simulink model "ServoCalibration"  (R2021b)
settings: Solver=FixedStepAuto  StartTime=0.0  StopTime=600  RelTol=1e-3  EnableMultiTasking=on
InitFcn:
  | hardwareSetup;
model workspace (MAT data in the model file):
  Ts_DynSim = Simulink.Parameter
  Ts_DynSim.Value = 0.005
  Ts_DynSim.DataType = 'auto'
  Ts_DynSim.Complexity = 'real'
  Ts_DynSim.Dimensions = [1 1]
values from neighbouring files (symbols this model uses):
  Ts_DynSim = 0.005    [MPCGen_OffsetFree.m]    (also in MPCGen_OffsetFree_UD.m; MPCGen_OffsetFree_estDis.m = 0.006; MPCcontrollerGen_OffsetFree.m; MPCcontrollerGen_OffsetFree_UD.m)
libraries: PuppyLibrary x5, simulink_extras x2
settings Model: SimulationMode=external  ExtModeTrigDuration=2  Creator=MSI-NB  LastModifiedBy=MSI-NB
settings SolverCC: AlgebraicLoopSolver=TrustRegion  PositivePriorityOrder=on
settings DataIOCC: ReturnWorkspaceOutputs=off
settings OptimizationCC: MaxStackSize=64
settings DebuggingCC: ParameterTunabilityLossMsg=error  SFMachineParentedDataDiag=warning  ArithmeticOperatorsInVariantConditions=warning
settings HardwareCC: ProdBitPerPointer=32  ProdBitPerSizeT=32  ProdBitPerPtrDiffT=32  ProdLargestAtomicInteger=Long  ProdLargestAtomicFloat=Double  ProdWordSize=32  ProdHWDeviceType=ARM Compatible->ARM Cortex  UseEmbeddedCoderFeatures=off
settings SFSimCC: SimUseLocalCustomCode=off  CustomCodeUndefinedFunction=UseInterfaceOnly
settings RTWCC: Description=Embedded Coder  SystemTargetFile=ert.tlc  HardwareBoard=Raspberry Pi  TLCOptions="-aInlineSetEventsForThisBaseRateFcn=TLC_FALSE -aSuppressMultiTaskScheduler=TLC_FALSE  -aRateBasedStepFcn=0"  TemplateMakefile=ert_default_tmf  RTWUseLocalCustomCode=off  Toolchain=GNU GCC Embedded Linux  BuildConfiguration=Faster Runs
settings CodeAppCC: ForceParamTrailComments=on  OperatorAnnotations=on  StateflowObjectComments=on  MATLABSourceComments=on
settings ERTTargetCC: ERTCustomFileBanners=off  SupportContinuousTime=on  SupportNonInlinedSFcns=on  RemoveResetFunc=off  SupportVariableSizeSignals=on  ModelStepFunctionPrototypeControlCompliant=off

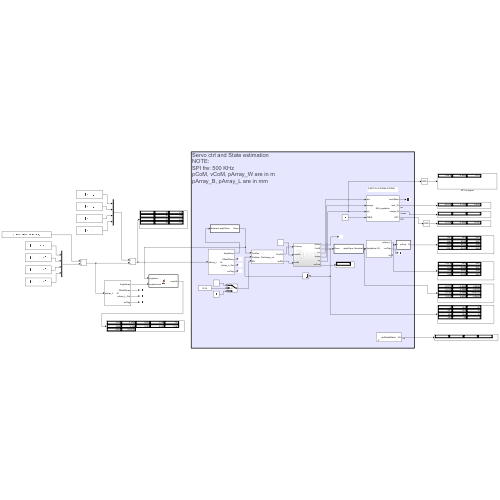
[thumbnail: Simulink's stored preview of the top-level diagram]
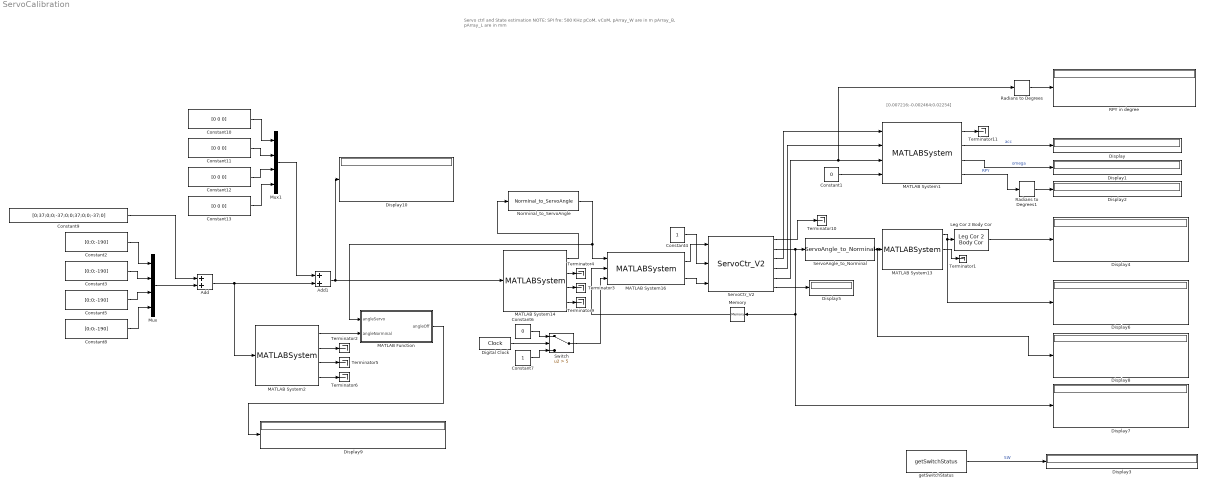
== system ServoCalibration ==
  note: [0.007216;-0.002464;0.02254]
  note: Servo ctrl and State estimation
      | NOTE:
      | SPI fre: 500 KHz
      | pCoM, vCoM, pArray_W are in m
      | pArray_B, pArray_L are in mm
  Add : Sum
  Add1 : Sum
  Constant1 : Constant  Value=0
  Constant{10..13} (4 alike) : Constant  Value=[0 0 0]
  Constant{2..3,5,8} (4 alike) : Constant  Value=[0;0;-190]
  Constant4 : Constant
  Constant6 : Constant  Value=0
  Constant7 : Constant
  Constant9 : Constant  Value=[0;37;0;0;-37;0;0;37;0;0;-37;0]
  Digital Clock : DigitalClock  SampleTime=Ts_DynSim
  Display{,1..10} (11 alike) : Display
  Leg Cor 2 Body Cor : PuppyLibrary/Leg Cor 2 Body Cor  SystemSampleTime=-1  VariantActivationTime=update diagram  Latency=0  AutoFrameSizeCalculation=off
  MATLAB Function : MATLAB Function  TreatAsAtomicUnit=on
  MATLAB System1 : MATLABSystem  System=IMU_regulation  pitOff=-0.4  rollOff=1  SimulateUsing=Code generation
      mask Type: IMU_regulation
      mask Display:
      | disp('IMU_regulation');
      | port_label('input',1,'acc');
      | port_label('input',2,'omega');
      | port_label('input',3,'rpy');
      | port_label('input',4,'OffEN');
      | port_label('output',1,'accOffnow');
      | port_label('output',2,'accL_W');
      | port_label('output',3,'omega_W');
      | port_label('output',4,'RPY');
  MATLAB System13 : MATLABSystem  System=FK  dt=0.005  SimulateUsing=Code generation
      mask Type: FK
      mask Display:
      | disp('FK');
      | port_label('input',1,'AngleArray');
      | port_label('output',1,'pArray_L');
      | port_label('output',2,'errFlag');
      | port_label('output',3,'dq');
  MATLAB System14 : MATLABSystem  System=IK  LF_Off=[ 0; 0; 0 ]  RF_Off=[ 0; 0; 0 ]  LH_Off=[ 0; 0; 0 ]  RH_Off=[ 0; 0; 0 ]  SimulateUsing=Code generation
      mask Type: IK
      mask Display:
      | disp('IK');
      | port_label('input',1,'pArray_L');
      | port_label('output',1,'AngleArray');
      | port_label('output',2,'OffsetPArray');
      | port_label('output',3,'pArray_L_Out');
      | port_label('output',4,'errFlag');
  MATLAB System16 : MATLABSystem  System=PosAssign_vel  cons_Vel=15  dt=Ts_DynSim  SimulateUsing=Code generation
      mask Type: PosAssign_vel
      mask Display:
      | disp('PosAssign_vel');
      | port_label('input',1,'PosDes');
      | port_label('input',2,'PosNow');
      | port_label('input',3,'EN');
      | port_label('output',1,'PosOut');
      | port_label('output',2,'setEN');
  MATLAB System2 : MATLABSystem  System=IK  LF_Off=[ 0; 0; 0 ]  RF_Off=[ 0; 0; 0 ]  LH_Off=[ 0; 0; 0 ]  RH_Off=[ 0; 0; 0 ]  SimulateUsing=Code generation
      mask Type: IK
      mask Display:
      | disp('IK');
      | port_label('input',1,'pArray_L');
      | port_label('output',1,'AngleArray');
      | port_label('output',2,'OffsetPArray');
      | port_label('output',3,'pArray_L_Out');
      | port_label('output',4,'errFlag');
  Memory : Memory  InitialCondition=zeros(12,1)
  Mux : Mux
  Mux1 : Mux
  Norminal_to_ServoAngle : PuppyLibrary/Norminal_to_ServoAngle  SystemSampleTime=-1  VariantActivationTime=update diagram  Latency=0  AutoFrameSizeCalculation=off
  RPY in degree : Display
  Radians to Degrees : simulink_extras/Transformations/Radians to Degrees
  Radians to Degrees1 : simulink_extras/Transformations/Radians to Degrees
  ServoAngle_to_Norminal : PuppyLibrary/ServoAngle_to_Norminal  SystemSampleTime=-1  VariantActivationTime=update diagram  Latency=0  AutoFrameSizeCalculation=off
  ServoCtr_V2 : PuppyLibrary/ServoCtr_V2  SystemSampleTime=-1  VariantActivationTime=update diagram  Latency=0  AutoFrameSizeCalculation=off
  Switch : Switch  Criteria=u2 > Threshold  Threshold=5
  Terminator{1..6,9..11} (9 alike) : Terminator
  getSwitchStatus : PuppyLibrary/getSwitchStatus  sampleTime=Ts_DynSim
  wires:
  Add/1 -> Add1/2, MATLAB System2/1
  MATLAB System14/1 -> Norminal_to_ServoAngle/1
  MATLAB System1/1 -> Terminator11/1
  MATLAB System16/1 -> ServoCtr_V2/1
  Constant9/1 -> Add/1
  MATLAB System16/2 -> ServoCtr_V2/3
  getSwitchStatus/1 -> Display3/1  "SW"
  MATLAB System13/2 -> Terminator1/1
  Constant7/1 -> Switch/3
  Constant1/1 -> MATLAB System1/4
  MATLAB System13/1 -> Display6/1, Leg Cor 2 Body Cor/1
  ServoCtr_V2/5 -> Radians to Degrees/1, MATLAB System1/3
  Leg Cor 2 Body Cor/1 -> Display4/1
  Digital Clock/1 -> Switch/2
  Switch/1 -> MATLAB System16/3
  ServoCtr_V2/6 -> Display5/1
  Memory/1 -> MATLAB System16/2
  ServoCtr_V2/2 -> Display7/1, Memory/1, ServoAngle_to_Norminal/1
  Constant5/1 -> Mux/3
  Constant4/1 -> ServoCtr_V2/2
  ServoAngle_to_Norminal/1 -> Display8/1, MATLAB System13/1
  MATLAB System1/2 -> Display/1  "acc"
  MATLAB System14/4 -> Terminator9/1
  MATLAB System1/4 -> Radians to Degrees1/1  "RPY"
  ServoCtr_V2/1 -> Terminator10/1
  Constant3/1 -> Mux/2
  ServoCtr_V2/3 -> MATLAB System1/1
  Constant2/1 -> Mux/1
  Radians to Degrees/1 -> RPY in degree/1
  Constant8/1 -> Mux/4
  MATLAB System1/3 -> Display1/1  "omega"
  MATLAB System14/3 -> Terminator3/1
  Constant6/1 -> Switch/1
  Mux/1 -> Add/2
  Norminal_to_ServoAngle/1 -> MATLAB Function/1(angleServo), MATLAB System16/1
  ServoCtr_V2/4 -> MATLAB System1/2
  MATLAB System2/3 -> Terminator5/1
  MATLAB System2/4 -> Terminator6/1
  Add1/1 -> MATLAB System14/1, Display10/1
  Constant12/1 -> Mux1/3
  Mux1/1 -> Add1/1
  Constant10/1 -> Mux1/1
  Constant11/1 -> Mux1/2
  Constant13/1 -> Mux1/4
  MATLAB System2/1 -> MATLAB Function/2(angleNorminal)
  MATLAB Function/1(angleOff) -> Display9/1
  MATLAB System2/2 -> Terminator2/1
  MATLAB System14/2 -> Terminator4/1
  Radians to Degrees1/1 -> Display2/1

== matlab function ServoCalibration/MATLAB Function ==
  data: angleServo input; angleOff output; angleNorminal input
function angleOff = fcn(angleServo,angleNorminal)
% extract angleOff from angleServo and angleNorminal

% angleNorminal: [12,1] vector, unit is radiuns, 
% counter clock-wise rotation, results direct from IK.
% angleServo: [12,1] vector, output to servos, labels should be [11,12,13,...,41,42,43]
% clock-wise position rotation, unit is degree
% angleOff: [12 1] vector, degree

%angleOff=[-8;0;-7;-7;-1;4;3;5;6;3;-5;2];

angleServoOri = angleNorminal/pi*180;
angleServoOri(9)=-angleServoOri(9);
angleServoOri(12)=-angleServoOri(12);
% for current servos, clock-wise rotation is the position direction
angleServoOri=-angleServoOri;

angleOff=angleServo-angleServoOri;
